simulink model "AC"  (R2020b)
settings: Solver=VariableStepAuto  StartTime=0.0  StopTime=10.0  RelTol=1e-3
undefined symbols (not defined in the file): c, M, Mdot
settings Model: Creator=xinbo  LastModifiedBy=xinbo

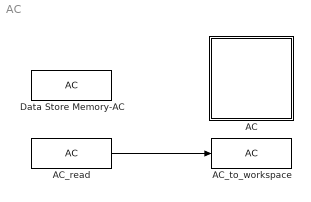
== system AC ==
  AC : Subsystem
      mask Display: image('/Users/xinbo/E/paper3/program_clean/digital_twin/images/AC.png'); % Use "Edit Image" on toolstrip to change.
  AC_read : DataStoreRead  DataStoreName=AC
  AC_to_workspace : ToWorkspace  VariableName=AC  SampleTime=-1
      settings: Save2DSignal=2-D array (concatenate along first dimension)
  Data Store Memory-AC : DataStoreMemory  DataStoreName=AC  ReadBeforeWriteMsg=warning  WriteAfterWriteMsg=warning  WriteAfterReadMsg=warning  ShowAdditionalParam=off  OutDataTypeStr=double
  wires:
  AC_read/1 -> AC_to_workspace/1

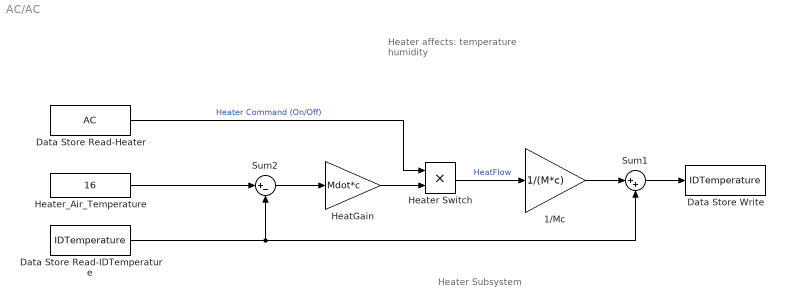
== system AC/AC ==
  note: Heater affects:
      | temperature
      | humidity
  note: Heater Subsystem
  1/Mc : Gain  Gain=1/(M*c)  SaturateOnIntegerOverflow=on  OutDataTypeStr=Inherit: Same as input  ParamDataTypeStr=Inherit: Same as input
  Data Store Read-Heater : DataStoreRead  DataStoreName=AC
  Data Store Read-IDTemperature : DataStoreRead  DataStoreName=IDTemperature
  Data Store Write : DataStoreWrite  DataStoreName=IDTemperature
  HeatGain : Gain  Gain=Mdot*c
  Heater Switch : Product  RndMeth=Zero
  Heater_Air_Temperature : Constant  Value=16
  Sum1 : Sum  Inputs=|++  InputSameDT=on  SaturateOnIntegerOverflow=on  OutDataTypeStr=Inherit: Same as first input
  Sum2 : Sum  Inputs=|+-
  wires:
  Data Store Read-Heater/1 -> Heater Switch/1  "Heater Command (On/Off)"
  Sum2/1 -> HeatGain/1
  Heater_Air_Temperature/1 -> Sum2/1
  HeatGain/1 -> Heater Switch/2
  Heater Switch/1 -> 1/Mc/1  "HeatFlow"
  1/Mc/1 -> Sum1/1
  Data Store Read-IDTemperature/1 -> Sum1/2, Sum2/2
  Sum1/1 -> Data Store Write/1
